simulink model "MSFartoystyring18"  (R2017b)
settings: Solver=ode45  StartTime=tstart  StopTime=tstop  RelTol=1e-3  EnableMultiTasking=on
values from neighbouring files (symbols this model uses):
  c = 1    [run22.m]    (also in run23.m)
  d1 = -0.0021    [init_controllers.m]    (also in run23.m = double(sol.d1))
  d2 = 1.0377    [init_controllers.m]    (also in run23.m = double(sol.d2))
  K = 0.0322    [init_controllers.m]    (also in run_task_1_2.m = x(2))
  Kd = 3*lambda_heading    (= 0.75)    [init_controllers.m]    (also in run23.m)
  Ki = lambda_heading^3    (= 0.015625)    [init_controllers.m]    (also in run23.m)
  Ki_speed = lambda_speed^2    (= 0.09)    [init_controllers.m]    (also in run23.m)
  Kp = 3*lambda_heading^2    (= 0.1875)    [init_controllers.m]    (also in run23.m)
  Kp_speed = 2*lambda_speed    (= 0.6)    [init_controllers.m]    (also in run23.m)
  m = 5550    [init_controllers.m]    (also in run23.m)
  omega_n = 0.008    [init_controllers.m]    (also in run23.m)
  p0 = [1500 500]    [run22.m]    (also in run23.m = zeros(2,1))
  psi0 = 50*deg2rad    (= 0.872664625997)    [run22.m]    (also in run23.m = 0)
  r0 = 0    [run22.m]    (also in run23.m)
  T = 65.6949    [init_controllers.m]    (also in run_task_1_2.m = 1/x(1))
  tsamp = 10    [run22.m]    (also in run23.m)
  u_r_0 = 100    [init_controllers.m]    (also in run23.m = 4)
  u_r_final = 100    [init_controllers.m]    (also in run23.m = 7)
  u_r_step_time = 2000    [init_controllers.m]    (also in run23.m = 500)
  v0 = [6.63 0]'    [run22.m]    (also in run23.m = [4 0]')
  zeta = 1    [run23.m]
undefined symbols (not defined in the file or in its folder): msfartoystyring
settings Model: ExtModeAutoUpdateStatusClock=off  Creator=christh  LastModifiedBy=henningward
settings DataIOCC: LimitDataPoints=on  SaveFormat=Array  SignalLoggingSaveFormat=ModelDataLogs
settings OptimizationCC: ExpressionDepthLimit=2147483647  InitFltsAndDblsToZero=on  LifeSpan=inf
settings DebuggingCC: UnderspecifiedInitializationDetection=Classic  MergeDetectMultiDrivingBlocksExec=none  SolverPrmCheckMsg=warning  FcnCallInpInsideContextMsg=warning  StateNameClashWarn=warning  SFUnexpectedBacktrackingDiag=warning  SFNoUnconditionalDefaultTransitionDiag=warning  SFExecutionAtInitializationDiag=none
settings HardwareCC: ProdBitPerPointer=32  ProdBitPerSizeT=32  ProdBitPerPtrDiffT=32  ProdLargestAtomicFloat=None  ProdIntDivRoundTo=Undefined  ProdEndianess=Unspecified  ProdWordSize=32  ProdHWDeviceType=32-bit Generic
settings ModelReferenceCC: PropagateSignalLabelsOutOfModel=off
settings CodeAppCC: StateflowObjectComments=on
settings GRTTargetCC: TargetLangStandard=C89/C90 (ANSI)  GeneratePreprocessorConditionals=Disable all  CombineOutputUpdateFcns=off  GRTInterface=on
settings ConfigComp: CovMetricSettings=dw  CovHtmlReporting=on  CovSaveCumulativeToWorkspaceVar=on  CovSaveSingleToWorkspaceVar=on  CovExternalEMLEnable=off

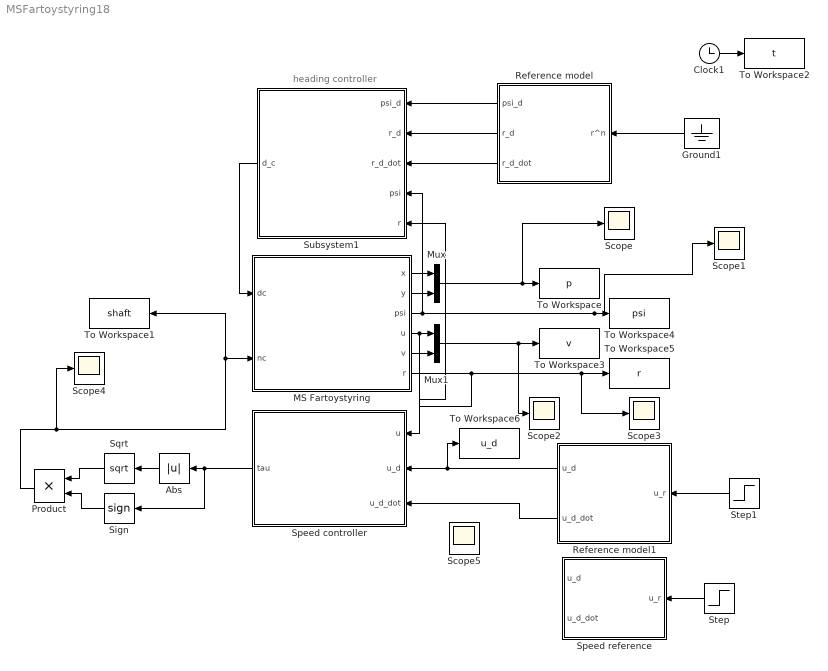
== system MSFartoystyring18 ==
  note: heading controller
  Abs : Abs
  Clock1 : Clock
  Ground1 : Ground
  MS Fartoystyring : Subsystem  mask(MS Fartoystyring for Assignment 3 G&C){x0=p0(1), y0=p0(2), u0=v0(1), v0=v0(2), psi0=psi0, r0=r0, c=c}
      mask prompts: x0 "x(t0) (m)"; y0 "y(t0) (m)"; u0 "u(t0) (m/s)"; v0 "v(t0) (m/s)"; psi0 "psi(t0) (rad)"; r0 "r(t0) (rad/s)"; c "current (0 or 1)"
      mask help:
      | Block corresponding to Figure 1 in the assignment text. Gives the response of the ship.
      |
      | The design speed of MS Fartoystyring is u=8.23 m/s.
      |
      | Input:
      | dc: commanded rudder (rad), dmax=25*pi/180
      | nc: commanded shaft speed (rad/s), nmax=85*2*pi/60
      |
      | Output:
      | x: north pos (m)
      | y: east pos (m)
      | u: surge (m/s)
      | v: sway (m/s)
      | psi: heading (rad)
      | r: yaw (rad/s)
      mask Help: Comments, bugs and help requests can be directed to the TA. Email on course website.
  Mux : Mux  Inputs=2
  Mux1 : Mux  Inputs=2
  Product : Product
  Reference model : Subsystem
  Reference model1 : Subsystem
  Scope{,1..5} (6 alike) : Scope
  Sign : Signum
  Speed controller : Subsystem
  Speed reference : Subsystem
  Sqrt : Sqrt  SaturateOnIntegerOverflow=on
  Step : Step  Time=u_r_step_time  Before=u_r_0  After=u_r_final  SampleTime=0
  Step1 : Step  Time=u_r_step_time  Before=u_r_0  After=u_r_final  SampleTime=tsamp
  Subsystem1 : Subsystem
  To Workspace : ToWorkspace  VariableName=p  SampleTime=tsamp
  To Workspace1 : ToWorkspace  VariableName=shaft  SampleTime=tsamp
  To Workspace2 : ToWorkspace  VariableName=t  SampleTime=tsamp
  To Workspace3 : ToWorkspace  VariableName=v  SampleTime=tsamp
  To Workspace4 : ToWorkspace  VariableName=psi  SampleTime=tsamp
  To Workspace5 : ToWorkspace  VariableName=r  SampleTime=tsamp
  To Workspace6 : ToWorkspace  VariableName=u_d  SampleTime=tsamp
  wires:
  MS Fartoystyring/1(x) -> Mux/1
  MS Fartoystyring/2(y) -> Mux/2
  MS Fartoystyring/4(u) -> Speed controller/1("u "), Mux1/1
  MS Fartoystyring/5(v) -> Mux1/2
  Mux/1 -> Scope/1, To Workspace/1
  Mux1/1 -> Scope2/1, To Workspace3/1
  MS Fartoystyring/6(r) -> Subsystem1/5(r), Scope3/1, To Workspace5/1
  Subsystem1/1("d_c ") -> MS Fartoystyring/1(dc)
  Clock1/1 -> To Workspace2/1
  Speed controller/1("tau ") -> Sign/1, Abs/1
  Abs/1 -> Sqrt/1
  Sign/1 -> Product/2
  Sqrt/1 -> Product/1
  Product/1 -> Scope4/1, To Workspace1/1, MS Fartoystyring/2(nc)
  Ground1/1 -> Reference model/1(r^n)
  Reference model/2(r_d) -> Subsystem1/2(r_d)
  Reference model/1(psi_d) -> Subsystem1/1(psi_d)
  Reference model/3(r_d_dot) -> Subsystem1/3(r_d_dot)
  MS Fartoystyring/3(psi) -> Scope1/1, To Workspace4/1, Subsystem1/4("psi ")
  Step1/1 -> Reference model1/1(u_r)
  Step/1 -> Speed reference/1(u_r)
  Reference model1/1(u_d) -> To Workspace6/1, Speed controller/2(u_d)
  Reference model1/2(u_d_dot) -> Speed controller/3(u_d_dot)

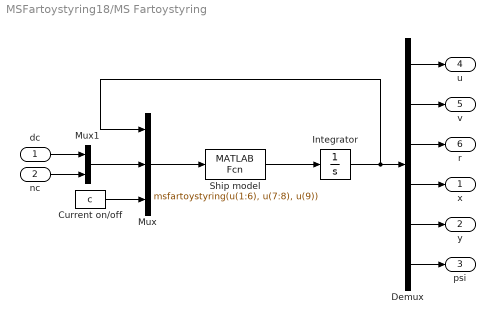
== system MSFartoystyring18/MS Fartoystyring ==
  dc : Inport
  nc : Inport  Port=2
  Current on/off : Constant  Value=c
  Demux : Demux  Outputs=6
  Integrator : Integrator  InitialCondition=[u0 v0 r0 x0 y0 psi0]'
  Mux : Mux  Inputs=3
  Mux1 : Mux  Inputs=2
  Ship model : MATLABFcn  MATLABFcn=msfartoystyring(u(1:6), u(7:8), u(9))  OutputDimensions=6
  x : Outport
  y : Outport  Port=2
  psi : Outport  Port=3
  u : Outport  Port=4
  v : Outport  Port=5
  r : Outport  Port=6
  wires:
  Integrator/1 -> Mux/1, Demux/1
  Mux1/1 -> Mux/2
  dc/1 -> Mux1/1
  nc/1 -> Mux1/2
  Demux/1 -> u/1
  Demux/2 -> v/1
  Demux/3 -> r/1
  Demux/4 -> x/1
  Demux/5 -> y/1
  Demux/6 -> psi/1
  Current on/off/1 -> Mux/3
  Ship model/1 -> Integrator/1
  Mux/1 -> Ship model/1

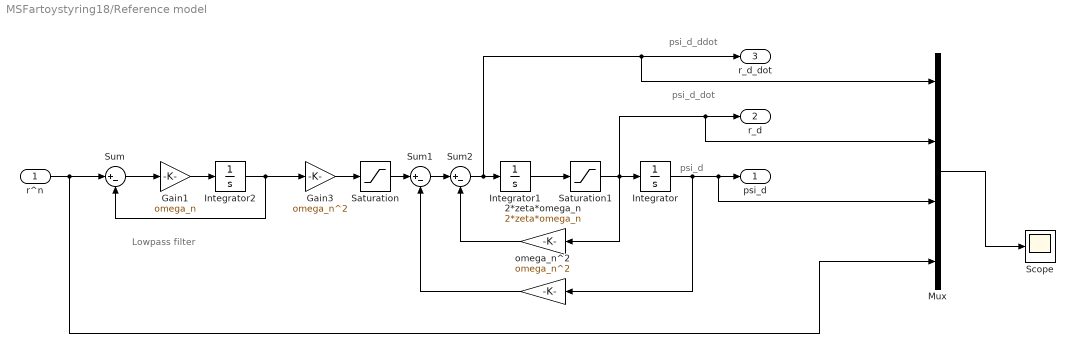
== system MSFartoystyring18/Reference model ==
  note: psi_d_ddot
  note: psi_d_dot
  note: Lowpass filter
  note: psi_d
  r^n : Inport
  2*zeta*omega_n : Gain  Gain=2*zeta*omega_n
  Gain1 : Gain  Gain=omega_n
  Gain3 : Gain  Gain=omega_n^2
  Integrator : Integrator
  Integrator1 : Integrator
  Integrator2 : Integrator
  Mux : Mux
  Saturation : Saturate  UpperLimit=1000  LowerLimit=-1000
  Saturation1 : Saturate  UpperLimit=1000  LowerLimit=-1000
  Scope : Scope
  Sum : Sum  Inputs=|+-
  Sum1 : Sum  Inputs=|+-
  Sum2 : Sum  Inputs=|+-
  omega_n^2 : Gain  Gain=omega_n^2
  psi_d : Outport
  r_d : Outport  Port=2
  r_d_dot : Outport  Port=3
  wires:
  Integrator1/1 -> Saturation1/1
  Saturation1/1 -> Mux/2, r_d/1, 2*zeta*omega_n/1, Integrator/1
  2*zeta*omega_n/1 -> Sum2/2
  Sum2/1 -> Mux/1, r_d_dot/1, Integrator1/1
  omega_n^2/1 -> Sum1/2
  Saturation/1 -> Sum1/1
  Gain3/1 -> Saturation/1
  Sum1/1 -> Sum2/1
  Sum/1 -> Gain1/1
  Integrator2/1 -> Sum/2, Gain3/1
  Gain1/1 -> Integrator2/1
  Integrator/1 -> Mux/3, psi_d/1, omega_n^2/1
  r^n/1 -> Mux/4, Sum/1
  Mux/1 -> Scope/1

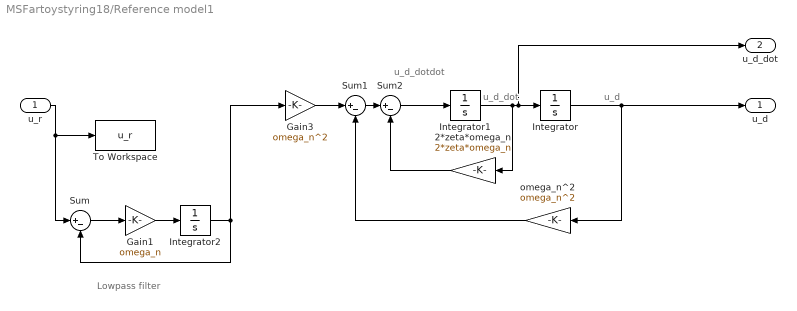
== system MSFartoystyring18/Reference model1 ==
  note: u_d
  note: u_d_dot
  note: u_d_dotdot
  note: Lowpass filter
  u_r : Inport
  2*zeta*omega_n : Gain  Gain=2*zeta*omega_n
  Gain1 : Gain  Gain=omega_n
  Gain3 : Gain  Gain=omega_n^2
  Integrator : Integrator  InitialCondition=u_r_0
  Integrator1 : Integrator
  Integrator2 : Integrator
  Sum : Sum  Inputs=|+-
  Sum1 : Sum  Inputs=|+-
  Sum2 : Sum  Inputs=|+-
  To Workspace : ToWorkspace  VariableName=u_r  SampleTime=-1
  omega_n^2 : Gain  Gain=omega_n^2
  u_d : Outport
  u_d_dot : Outport  Port=2
  wires:
  Integrator1/1 -> 2*zeta*omega_n/1, Integrator/1, u_d_dot/1
  2*zeta*omega_n/1 -> Sum2/2
  Sum1/1 -> Sum2/1
  omega_n^2/1 -> Sum1/2
  Gain3/1 -> Sum1/1
  Sum2/1 -> Integrator1/1
  Integrator/1 -> omega_n^2/1, u_d/1
  Gain1/1 -> Integrator2/1
  Sum/1 -> Gain1/1
  u_r/1 -> To Workspace/1, Sum/1
  Integrator2/1 -> Gain3/1, Sum/2

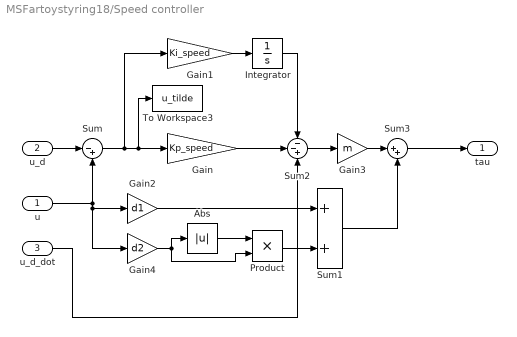
== system MSFartoystyring18/Speed controller ==
  "u " : Inport
  u_d : Inport  Port=2
  u_d_dot : Inport  Port=3
  Abs : Abs
  Gain : Gain  Gain=Kp_speed
  Gain1 : Gain  Gain=Ki_speed
  Gain2 : Gain  Gain=d1
  Gain3 : Gain  Gain=m
  Gain4 : Gain  Gain=d2
  Integrator : Integrator
  Product : Product
  Sum : Sum  Inputs=|-+
  Sum1 : Sum
  Sum2 : Sum  Inputs=--+
  Sum3 : Sum  Inputs=|++
  To Workspace3 : ToWorkspace  VariableName=u_tilde  SampleTime=tsamp
  "tau " : Outport
  wires:
  Integrator/1 -> Sum2/1
  Gain/1 -> Sum2/2
  Sum2/1 -> Gain3/1
  Gain3/1 -> Sum3/1
  u_d_dot/1 -> Sum2/3
  Sum/1 -> To Workspace3/1, Gain/1, Gain1/1
  Gain1/1 -> Integrator/1
  u_d/1 -> Sum/1
  "u "/1 -> Gain4/1, Gain2/1, Sum/2
  Abs/1 -> Product/1
  Gain4/1 -> Abs/1, Product/2
  Gain2/1 -> Sum1/1
  Product/1 -> Sum1/2
  Sum1/1 -> Sum3/2
  Sum3/1 -> "tau "/1

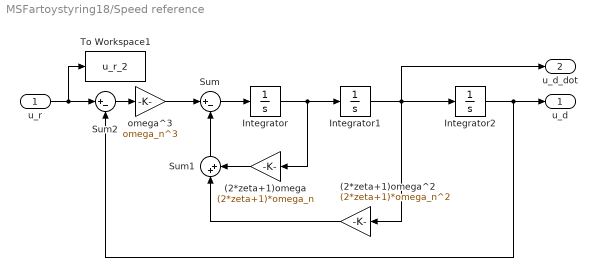
== system MSFartoystyring18/Speed reference ==
  u_r : Inport
  (2*zeta+1)omega : Gain  Gain=(2*zeta+1)*omega_n
  (2*zeta+1)omega^2 : Gain  Gain=(2*zeta+1)*omega_n^2
  Integrator : Integrator
  Integrator1 : Integrator
  Integrator2 : Integrator  InitialCondition=u_r_0
  Sum : Sum  Inputs=|+-
  Sum1 : Sum  Inputs=|++
  Sum2 : Sum  Inputs=|+-
  To Workspace1 : ToWorkspace  VariableName=u_r_2  SampleTime=tsamp
  omega^3 : Gain  Gain=omega_n^3
  u_d : Outport
  u_d_dot : Outport  Port=2
  wires:
  Integrator2/1 -> Sum2/2, u_d/1
  Integrator/1 -> Integrator1/1, (2*zeta+1)omega/1
  Integrator1/1 -> (2*zeta+1)omega^2/1, u_d_dot/1, Integrator2/1
  omega^3/1 -> Sum/1
  Sum/1 -> Integrator/1
  Sum1/1 -> Sum/2
  (2*zeta+1)omega^2/1 -> Sum1/1
  (2*zeta+1)omega/1 -> Sum1/2
  Sum2/1 -> omega^3/1
  u_r/1 -> To Workspace1/1, Sum2/1

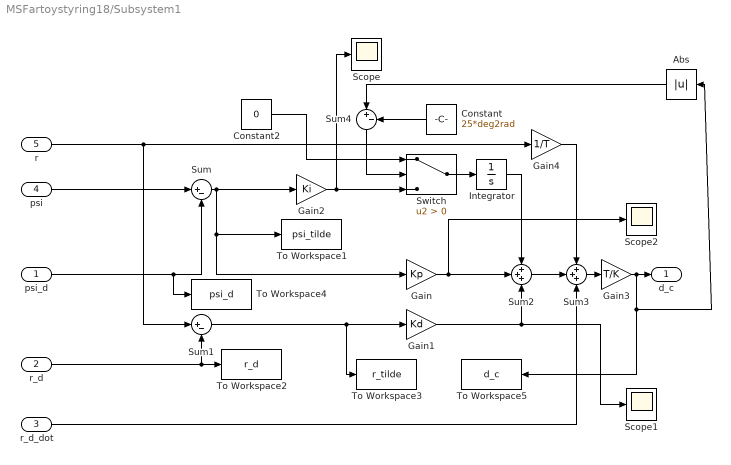
== system MSFartoystyring18/Subsystem1 ==
  psi_d : Inport
  r_d : Inport  Port=2
  r_d_dot : Inport  Port=3
  "psi " : Inport  Port=4
  r : Inport  Port=5
  Abs : Abs
  Constant : Constant  Value=25*deg2rad
  Constant2 : Constant  Value=0
  Gain : Gain  Gain=Kp
  Gain1 : Gain  Gain=Kd
  Gain2 : Gain  Gain=Ki
  Gain3 : Gain  Gain=T/K
  Gain4 : Gain  Gain=1/T
  Integrator : Integrator
  Scope : Scope
  Scope1 : Scope
  Scope2 : Scope
  Sum : Sum  Inputs=|+-
  Sum1 : Sum  Inputs=|+-
  Sum2 : Sum  Inputs=+++
  Sum3 : Sum  Inputs=+++
  Sum4 : Sum  Inputs=|+-
  Switch : Switch  Criteria=u2 > Threshold
  To Workspace1 : ToWorkspace  VariableName=psi_tilde  SampleTime=tsamp
  To Workspace2 : ToWorkspace  VariableName=r_d  SampleTime=tsamp
  To Workspace3 : ToWorkspace  VariableName=r_tilde  SampleTime=tsamp
  To Workspace4 : ToWorkspace  VariableName=psi_d  SampleTime=tsamp
  To Workspace5 : ToWorkspace  VariableName=d_c  SampleTime=tsamp
  "d_c " : Outport
  wires:
  "psi "/1 -> Sum/1
  r_d/1 -> To Workspace2/1, Sum1/2
  Sum1/1 -> To Workspace3/1, Gain1/1
  Integrator/1 -> Sum2/1
  Sum/1 -> Gain/1, To Workspace1/1, Gain2/1
  Gain2/1 -> Switch/3, Scope/1
  Gain/1 -> Scope2/1, Sum2/2
  Gain1/1 -> Scope1/1, Sum2/3
  psi_d/1 -> To Workspace4/1, Sum/2
  Switch/1 -> Integrator/1
  Gain3/1 -> To Workspace5/1, Abs/1, "d_c "/1
  Sum3/1 -> Gain3/1
  Sum2/1 -> Sum3/2
  r/1 -> Sum1/1, Gain4/1
  Abs/1 -> Sum4/1
  Constant/1 -> Sum4/2
  Sum4/1 -> Switch/2
  Constant2/1 -> Switch/1
  Gain4/1 -> Sum3/1
  r_d_dot/1 -> Sum3/3
